simulink model "Basic_oneDOF_wave_variable_control"  (R2016a)
settings: Solver=VariableStepAuto  StartTime=0.0  StopTime=10.0  RelTol=1e-3
values from neighbouring files (symbols this model uses):
  b1 = b    (= 2.5)    [Tanner_Niemeyer_high_frequency_force_parameters.m]    (also in Tanner_Niemeyer_wave_filtering_parameters.m; Xizhe_wave_filtering_parameters.m = 300; Ye_Liu_augmented_trajectory_tracking_parameters.m; high_frequency_force_parameters.m = 300)
  b2 = sqrt(2*b)    [Tanner_Niemeyer_high_frequency_force_parameters.m]    (also in Tanner_Niemeyer_wave_filtering_parameters.m; Xizhe_wave_filtering_parameters.m; Ye_Liu_augmented_trajectory_tracking_parameters.m; high_frequency_force_parameters.m)
  b3 = sqrt(2/b)    [Tanner_Niemeyer_high_frequency_force_parameters.m]    (also in Tanner_Niemeyer_wave_filtering_parameters.m; Xizhe_wave_filtering_parameters.m; Ye_Liu_augmented_trajectory_tracking_parameters.m; high_frequency_force_parameters.m)
  b4 = 1/b    (= 0.4)    [Tanner_Niemeyer_high_frequency_force_parameters.m]    (also in Tanner_Niemeyer_wave_filtering_parameters.m; Xizhe_wave_filtering_parameters.m = 0.00333333333333; Ye_Liu_augmented_trajectory_tracking_parameters.m; high_frequency_force_parameters.m = 0.00333333333333)
  bm = 0.005    [Daniela_basic_parameters.m]    (also in Tanner_Niemeyer_high_frequency_force_parameters.m; Tanner_Niemeyer_wave_filtering_parameters.m; Xizhe_wave_filtering_parameters.m; Ye_Liu_augmented_trajectory_tracking_parameters.m = 2.5)
  bs = 0.005    [Daniela_basic_parameters.m]    (also in Tanner_Niemeyer_high_frequency_force_parameters.m; Tanner_Niemeyer_wave_filtering_parameters.m; Xizhe_wave_filtering_parameters.m; Ye_Liu_augmented_trajectory_tracking_parameters.m = 2.5)
  Jm = 1    [Daniela_basic_parameters.m]    (also in Tanner_Niemeyer_high_frequency_force_parameters.m = 0.1; Tanner_Niemeyer_wave_filtering_parameters.m = 0.1; Xizhe_wave_filtering_parameters.m; Ye_Liu_augmented_trajectory_tracking_parameters.m = 0.1)
  Js = 1    [Daniela_basic_parameters.m]    (also in Tanner_Niemeyer_high_frequency_force_parameters.m = 0.1; Tanner_Niemeyer_wave_filtering_parameters.m = 0.1; Xizhe_wave_filtering_parameters.m; Ye_Liu_augmented_trajectory_tracking_parameters.m = 0.1)
  Ki = 200    [Daniela_basic_parameters.m]    (also in Tanner_Niemeyer_high_frequency_force_parameters.m = 370; Tanner_Niemeyer_wave_filtering_parameters.m = 370; Xizhe_wave_filtering_parameters.m = 2000; Ye_Liu_augmented_trajectory_tracking_parameters.m = 370)
  Kp = 1    [Daniela_basic_parameters.m]    (also in Tanner_Niemeyer_high_frequency_force_parameters.m = 2.5; Tanner_Niemeyer_wave_filtering_parameters.m = 2.5; Xizhe_wave_filtering_parameters.m = 200; Ye_Liu_augmented_trajectory_tracking_parameters.m = 20)
  Td = 0.03    [Daniela_basic_parameters.m]    (also in Tanner_Niemeyer_high_frequency_force_parameters.m; Tanner_Niemeyer_wave_filtering_parameters.m = 0.1; Xizhe_wave_filtering_parameters.m; Ye_Liu_augmented_trajectory_tracking_parameters.m = 0.5)
  x_m0 = 0    [Daniela_basic_parameters.m]    (also in Tanner_Niemeyer_high_frequency_force_parameters.m; Tanner_Niemeyer_wave_filtering_parameters.m; Xizhe_wave_filtering_parameters.m; Ye_Liu_augmented_trajectory_tracking_parameters.m)
  x_s0 = 0    [Daniela_basic_parameters.m]    (also in Tanner_Niemeyer_high_frequency_force_parameters.m; Tanner_Niemeyer_wave_filtering_parameters.m; Xizhe_wave_filtering_parameters.m; Ye_Liu_augmented_trajectory_tracking_parameters.m)
  xdot_m0 = 0    [Daniela_basic_parameters.m]    (also in Tanner_Niemeyer_high_frequency_force_parameters.m; Tanner_Niemeyer_wave_filtering_parameters.m; Xizhe_wave_filtering_parameters.m; Ye_Liu_augmented_trajectory_tracking_parameters.m)
  xdot_s0 = 0    [Daniela_basic_parameters.m]    (also in Tanner_Niemeyer_high_frequency_force_parameters.m; Tanner_Niemeyer_wave_filtering_parameters.m; Xizhe_wave_filtering_parameters.m; Ye_Liu_augmented_trajectory_tracking_parameters.m)
libraries: simulink x4
settings Model: Creator=Administrator  LastModifiedBy=Administrator

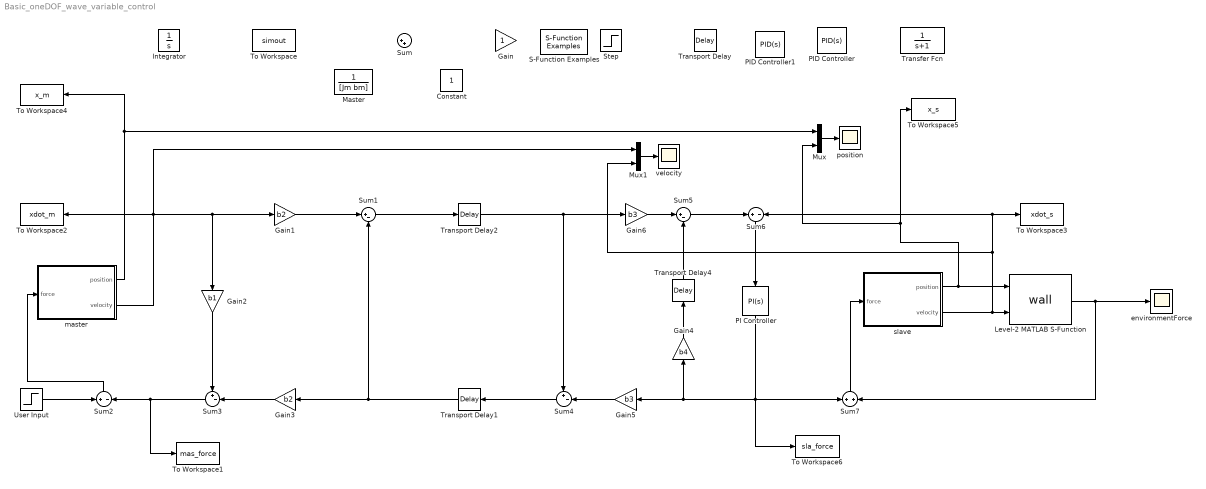
== system Basic_oneDOF_wave_variable_control ==
  Constant : Constant
  Gain : Gain
  Gain1 : Gain  Gain=b2
  Gain2 : Gain  Gain=b1
  Gain3 : Gain  Gain=b2
  Gain4 : Gain  Gain=b4
  Gain5 : Gain  Gain=b3
  Gain6 : Gain  Gain=b3
  Integrator : Integrator
  Level-2 MATLAB S-Function : M-S-Function  FunctionName=wall  Parameters=Kwall, bwall, xwall
  Master : TransferFcn  Denominator=[Jm bm]
  Mux : Mux  Inputs=2
  Mux1 : Mux  Inputs=2
  PI Controller : simulink/Continuous/PID Controller  Controller=PI  TimeDomain=Continuous-time  SampleTime=-1  IntegratorMethod=Forward Euler  FilterMethod=Forward Euler  Form=Parallel  UseFilter=on  ControllerParametersSource=internal  P=Kp  I=Ki  D=0  N=100  InitialConditionSource=internal  InitialConditionForIntegrator=0  InitialConditionForFilter=0  ExternalReset=none  LimitOutput=off  UpperSaturationLimit=inf  LowerSaturationLimit=-inf  LinearizeAsGain=on  AntiWindupMode=none  Kb=1  TrackingMode=off  Kt=1  PParamMin=[]  PParamMax=[]  IParamMin=[]  IParamMax=[]  DParamMin=[]  DParamMax=[]  NParamMin=[]  NParamMax=[]  KbParamMin=[]  KbParamMax=[]  KtParamMin=[]  KtParamMax=[]  POutMin=[]  POutMax=[]  IOutMin=[]  IOutMax=[]  DOutMin=[]  DOutMax=[]  NOutMin=[]  NOutMax=[]  KbOutMin=[]  KbOutMax=[]  KtOutMin=[]  KtOutMax=[]  IntegratorOutMin=[]  IntegratorOutMax=[]  FilterOutMin=[]  FilterOutMax=[]  SumOutMin=[]  SumOutMax=[]  SumI1OutMin=[]  SumI1OutMax=[]  SumI2OutMin=[]  SumI2OutMax=[]  SumI3OutMin=[]  SumI3OutMax=[]  SumDOutMin=[]  SumDOutMax=[]  SaturationOutMin=[]  SaturationOutMax=[]  IntegratorContinuousStateAttributes=''  IntegratorStateMustResolveToSignalObject=off  IntegratorRTWStateStorageClass=Auto  FilterContinuousStateAttributes=''  FilterStateMustResolveToSignalObject=off  FilterRTWStateStorageClass=Auto  DifferentiatorICPrevScaledInput=0  DifferentiatorOutMin=[]  DifferentiatorOutMax=[]
  PID Controller : simulink/Continuous/PID Controller  Controller=PID  TimeDomain=Continuous-time  SampleTime=-1  IntegratorMethod=Forward Euler  FilterMethod=Forward Euler  Form=Parallel  UseFilter=on  ControllerParametersSource=internal  P=1  I=1  D=0  N=100  InitialConditionSource=internal  InitialConditionForIntegrator=0  InitialConditionForFilter=0  ExternalReset=none  LimitOutput=off  UpperSaturationLimit=inf  LowerSaturationLimit=-inf  LinearizeAsGain=on  AntiWindupMode=none  Kb=1  TrackingMode=off  Kt=1  PParamMin=[]  PParamMax=[]  IParamMin=[]  IParamMax=[]  DParamMin=[]  DParamMax=[]  NParamMin=[]  NParamMax=[]  KbParamMin=[]  KbParamMax=[]  KtParamMin=[]  KtParamMax=[]  POutMin=[]  POutMax=[]  IOutMin=[]  IOutMax=[]  DOutMin=[]  DOutMax=[]  NOutMin=[]  NOutMax=[]  KbOutMin=[]  KbOutMax=[]  KtOutMin=[]  KtOutMax=[]  IntegratorOutMin=[]  IntegratorOutMax=[]  FilterOutMin=[]  FilterOutMax=[]  SumOutMin=[]  SumOutMax=[]  SumI1OutMin=[]  SumI1OutMax=[]  SumI2OutMin=[]  SumI2OutMax=[]  SumI3OutMin=[]  SumI3OutMax=[]  SumDOutMin=[]  SumDOutMax=[]  SaturationOutMin=[]  SaturationOutMax=[]  IntegratorContinuousStateAttributes=''  IntegratorStateMustResolveToSignalObject=off  IntegratorRTWStateStorageClass=Auto  FilterContinuousStateAttributes=''  FilterStateMustResolveToSignalObject=off  FilterRTWStateStorageClass=Auto  DifferentiatorICPrevScaledInput=0  DifferentiatorOutMin=[]  DifferentiatorOutMax=[]
  PID Controller1 : simulink/Continuous/PID Controller  Controller=PID  TimeDomain=Continuous-time  SampleTime=-1  IntegratorMethod=Forward Euler  FilterMethod=Forward Euler  Form=Parallel  UseFilter=on  ControllerParametersSource=internal  P=1  I=1  D=0  N=100  InitialConditionSource=internal  InitialConditionForIntegrator=0  InitialConditionForFilter=0  ExternalReset=none  LimitOutput=off  UpperSaturationLimit=inf  LowerSaturationLimit=-inf  LinearizeAsGain=on  AntiWindupMode=none  Kb=1  TrackingMode=off  Kt=1  PParamMin=[]  PParamMax=[]  IParamMin=[]  IParamMax=[]  DParamMin=[]  DParamMax=[]  NParamMin=[]  NParamMax=[]  KbParamMin=[]  KbParamMax=[]  KtParamMin=[]  KtParamMax=[]  POutMin=[]  POutMax=[]  IOutMin=[]  IOutMax=[]  DOutMin=[]  DOutMax=[]  NOutMin=[]  NOutMax=[]  KbOutMin=[]  KbOutMax=[]  KtOutMin=[]  KtOutMax=[]  IntegratorOutMin=[]  IntegratorOutMax=[]  FilterOutMin=[]  FilterOutMax=[]  SumOutMin=[]  SumOutMax=[]  SumI1OutMin=[]  SumI1OutMax=[]  SumI2OutMin=[]  SumI2OutMax=[]  SumI3OutMin=[]  SumI3OutMax=[]  SumDOutMin=[]  SumDOutMax=[]  SaturationOutMin=[]  SaturationOutMax=[]  IntegratorContinuousStateAttributes=''  IntegratorStateMustResolveToSignalObject=off  IntegratorRTWStateStorageClass=Auto  FilterContinuousStateAttributes=''  FilterStateMustResolveToSignalObject=off  FilterRTWStateStorageClass=Auto  DifferentiatorICPrevScaledInput=0  DifferentiatorOutMin=[]  DifferentiatorOutMax=[]
  S-Function Examples : simulink/User-Defined Functions/S-Function Examples
  Step : Step  SampleTime=0
  Sum : Sum  Inputs=|++
  Sum1 : Sum  Inputs=|+-
  Sum2 : Sum  Inputs=+|-
  Sum3 : Sum  Inputs=+-|
  Sum4 : Sum  Inputs=+-|
  Sum5 : Sum  Inputs=|+-
  Sum6 : Sum  Inputs=+|-
  Sum7 : Sum  Inputs=+|+
  To Workspace : ToWorkspace  VariableName=simout  SaveFormat=Timeseries  SampleTime=-1
  To Workspace1 : ToWorkspace  VariableName=mas_force  SaveFormat=Timeseries  SampleTime=-1
  To Workspace2 : ToWorkspace  VariableName=xdot_m  SaveFormat=Timeseries  SampleTime=-1
  To Workspace3 : ToWorkspace  VariableName=xdot_s  SaveFormat=Timeseries  SampleTime=-1
  To Workspace4 : ToWorkspace  VariableName=x_m  SaveFormat=Timeseries  SampleTime=-1
  To Workspace5 : ToWorkspace  VariableName=x_s  SaveFormat=Timeseries  SampleTime=-1
  To Workspace6 : ToWorkspace  VariableName=sla_force  SaveFormat=Timeseries  SampleTime=-1
  Transfer Fcn : TransferFcn  Denominator=[1 1]
  Transport Delay : TransportDelay
  Transport Delay1 : TransportDelay  DelayTime=Td
  Transport Delay2 : TransportDelay  DelayTime=Td
  Transport Delay4 : TransportDelay  DelayTime=0.001
  User Input : Step  SampleTime=0
  environmentForce : Scope
  "master " : Subsystem
  position : Scope
  "slave " : Subsystem
  velocity : Scope
  wires:
  User Input/1 -> Sum2/1
  Sum3/1 -> To Workspace1/1, Sum2/2
  Gain2/1 -> Sum3/1
  Gain1/1 -> Sum1/1
  Gain3/1 -> Sum3/2
  Sum1/1 -> Transport Delay2/1
  Transport Delay2/1 -> Sum4/1, Gain6/1
  Sum4/1 -> Transport Delay1/1
  Transport Delay1/1 -> Sum1/2, Gain3/1
  Gain6/1 -> Sum5/1
  Gain4/1 -> Transport Delay4/1
  Gain5/1 -> Sum4/2
  Sum5/1 -> Sum6/1
  Sum7/1 -> "slave "/1(force)
  Sum6/1 -> PI Controller/1
  PI Controller/1 -> Sum7/1, Gain4/1, Gain5/1, To Workspace6/1
  Sum2/1 -> "master "/1(force)
  "master "/1("position ") -> Mux/1, To Workspace4/1
  "master "/2(velocity) -> Mux1/1, Gain2/1, Gain1/1, To Workspace2/1
  "slave "/1("position ") -> Level-2 MATLAB S-Function/1, To Workspace5/1, Mux/2
  "slave "/2(velocity) -> Level-2 MATLAB S-Function/2, Sum6/2, To Workspace3/1, Mux1/2
  Level-2 MATLAB S-Function/1 -> environmentForce/1, Sum7/2
  Mux/1 -> position/1
  Mux1/1 -> velocity/1
  Transport Delay4/1 -> Sum5/2

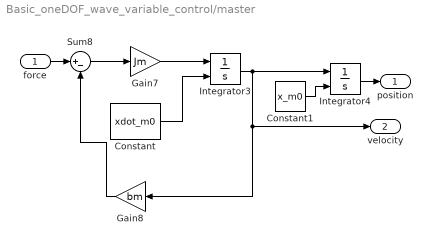
== system Basic_oneDOF_wave_variable_control/master  ==
  force : Inport
  Constant : Constant  Value=xdot_m0
  Constant1 : Constant  Value=x_m0
  Gain7 : Gain  Gain=Jm
  Gain8 : Gain  Gain=bm
  Integrator3 : Integrator  InitialConditionSource=external
  Integrator4 : Integrator  InitialConditionSource=external
  Sum8 : Sum  Inputs=|+-
  "position " : Outport
  velocity : Outport  Port=2
  wires:
  Integrator3/1 -> Integrator4/1, velocity/1, Gain8/1
  Sum8/1 -> Gain7/1
  Gain8/1 -> Sum8/2
  force/1 -> Sum8/1
  Integrator4/1 -> "position "/1
  Constant/1 -> Integrator3/2
  Constant1/1 -> Integrator4/2
  Gain7/1 -> Integrator3/1

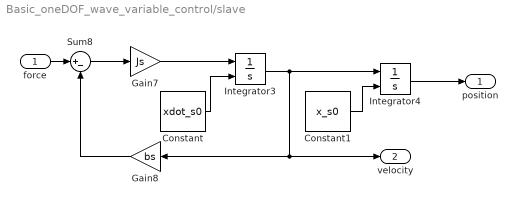
== system Basic_oneDOF_wave_variable_control/slave  ==
  force : Inport
  Constant : Constant  Value=xdot_s0
  Constant1 : Constant  Value=x_s0
  Gain7 : Gain  Gain=Js
  Gain8 : Gain  Gain=bs
  Integrator3 : Integrator  InitialConditionSource=external
  Integrator4 : Integrator  InitialConditionSource=external
  Sum8 : Sum  Inputs=|+-
  "position " : Outport
  velocity : Outport  Port=2
  wires:
  Integrator3/1 -> Integrator4/1, velocity/1, Gain8/1
  Sum8/1 -> Gain7/1
  Gain8/1 -> Sum8/2
  force/1 -> Sum8/1
  Integrator4/1 -> "position "/1
  Constant/1 -> Integrator3/2
  Gain7/1 -> Integrator3/1
  Constant1/1 -> Integrator4/2
